simulink model "con_act_atck"  (R2021a)
settings: Solver=VariableStepAuto  StartTime=0.0  StopTime=30.0  RelTol=1e-3
settings Model: Creator=Suman  LastModifiedBy=Suman

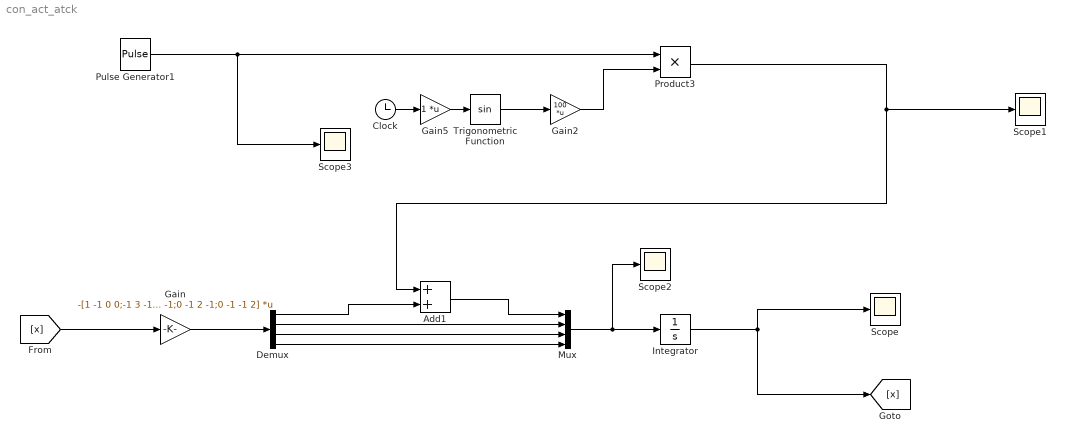
== system con_act_atck ==
  Add1 : Sum
  Clock : Clock
  Demux : Demux
  Gain : Gain  Gain=-[1 -1 0 0;-1 3 -1 -1;0 -1 2 -1;0 -1 -1 2]  Multiplication=Matrix(K*u) (u vector)
  Gain2 : Gain  Gain=100  Multiplication=Matrix(K*u) (u vector)
  Gain5 : Gain  Multiplication=Matrix(K*u) (u vector)
  Integrator : Integrator  InitialCondition=100*rand(4,1)
  Mux : Mux
  Product3 : Product
  Pulse Generator1 : DiscretePulseGenerator  PulseType=Time based  Period=30  PulseWidth=10  PhaseDelay=7
  Scope{,1..3} (4 alike) : Scope
  Trigonometric Function : Trigonometry
  wires:
  [x] -> Gain/1
  Pulse Generator1/1 -> Scope3/1, Product3/1
  Integrator/1 -> Scope/1, [x]
  Gain/1 -> Demux/1
  Product3/1 -> Scope1/1, Add1/1
  Gain5/1 -> Trigonometric Function/1
  Gain2/1 -> Product3/2
  Clock/1 -> Gain5/1
  Trigonometric Function/1 -> Gain2/1
  Add1/1 -> Mux/1
  Mux/1 -> Scope2/1, Integrator/1
  Demux/2 -> Mux/2
  Demux/3 -> Mux/3
  Demux/1 -> Add1/2
  Demux/4 -> Mux/4
